simulink model "Catwell_Rom"  (R2023a)
settings: Solver=FixedStepDiscrete  StartTime=0.0  StopTime=3.999  FixedStep=.01  RelTol=1e-3
libraries: Pathfinding_lib x4, simulink x2, embmathops x1, dspsigops x1, drivinglib x1
settings Model: SimulationMode=accelerator  Creator=FIRSTMentor  LastModifiedBy=ander

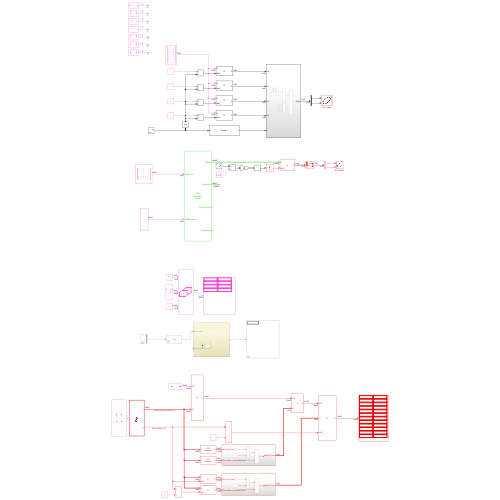
[thumbnail: Simulink's stored preview of the top-level diagram]
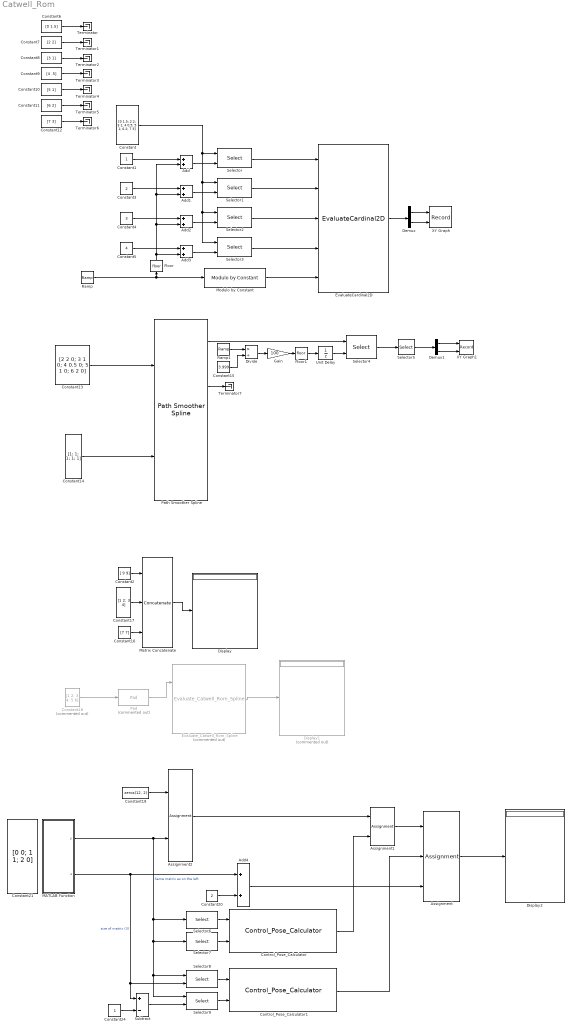
== system Catwell_Rom ==
  Add{,1..4} (5 alike) : Sum
  Assignment : Assignment  NumberOfDimensions=2  DiagnosticForDimensions=Warning  IndexOptions=Starting index (port),Assign all  Indices=1,1  OutputSizes=1,1
  Assignment1 : Assignment  NumberOfDimensions=2  DiagnosticForDimensions=Warning  IndexOptions=Starting index (dialog),Assign all  Indices=1,1  OutputSizes=1,1
  Assignment2 : Assignment  NumberOfDimensions=2  DiagnosticForDimensions=Warning  IndexOptions=Starting index (dialog),Assign all  Indices=2,2  OutputSizes=1,1
  Constant : Constant  Value=[0 1.5; 2 2; 3 1; 4 0.5; 5 1; 6 2; 7 3]  VectorParams1D=off
  Constant1 : Constant
  Constant10 : Constant  Value=[5 1]
  Constant11 : Constant  Value=[6 2]
  Constant12 : Constant  Value=[7 3]
  Constant13 : Constant  Value=[2 2 0; 3 1 0; 4 0.5 0; 5 1 0; 6 2 0]  VectorParams1D=off
  Constant14 : Constant  Value=[1; 1; 1; 1; 1]  VectorParams1D=off
  Constant15 : Constant  Value=3.999
  Constant16 : Constant  Value=[7 7]  VectorParams1D=off
  Constant17 : Constant  Value=[1 2; 3 4]  VectorParams1D=off
  Constant18 : Constant  Commented=on  Value=[1 2; 3 4; 5 6]
  Constant19 : Constant  Value=zeros(12, 2)
  Constant2 : Constant  Value=[ 9 9]  VectorParams1D=off
  Constant20 : Constant  Value=2
  Constant21 : Constant  Value=[0 0; 1 1; 2 0]
  Constant24 : Constant
  Constant3 : Constant  Value=2
  Constant4 : Constant  Value=3
  Constant5 : Constant  Value=4
  Constant6 : Constant  Value=[0 1.5]
  Constant7 : Constant  Value=[2 2]
  Constant8 : Constant  Value=[3 1]
  Constant9 : Constant  Value=[4 .5]
  Control_Pose_Calculator : Pathfinding_lib/Control_Pose_Calculator  SystemSampleTime=-1  VariantActivationTime=update diagram  Latency=0  AutoFrameSizeCalculation=off
  Control_Pose_Calculator1 : Pathfinding_lib/Control_Pose_Calculator  SystemSampleTime=-1  VariantActivationTime=update diagram  Latency=0  AutoFrameSizeCalculation=off
  Demux : Demux  Outputs=2
  Demux1 : Demux  Outputs=2
  Display : Display
  Display1 : Display  Commented=on
  Display2 : Display
  Divide : Product  Inputs=*/  RndMeth=Zero  SaturateOnIntegerOverflow=on
  EvaluateCardinal2D : Pathfinding_lib/EvaluateCardinal2D  SystemSampleTime=-1  VariantActivationTime=update diagram  Latency=0  AutoFrameSizeCalculation=off
  Evaluate_Catwell_Rom_Spline : Pathfinding_lib/Evaluate_Catwell_Rom_Spline  Commented=on  SystemSampleTime=-1  VariantActivationTime=update diagram  Latency=0  AutoFrameSizeCalculation=off
  Floor : Rounding
  Floor1 : Rounding
  Gain : Gain  Gain=100
  MATLAB Function : MATLAB Function  TreatAsAtomicUnit=on
  Matrix Concatenate : Concatenate  NumInputs=3  Mode=Multidimensional array
  Modulo by Constant : embmathops/Modulo by Constant  Denominator=1  SimulateUsing=Code generation
      settings: LibrarySourceBlock=embeddedMathLib/Modulo by Constant
  Pad : dspsigops/Pad  Commented=on  padAlong=Columns  dimsToPad=1  valSrc=Specify via dialog  padVal=-1  spec=Output size  padNumOutRowsSpecMethod=User-specified  numOutRows=Spline_Max_Num_RefPoses  padNumOutColsSpecMethod=User-specified  numOutCols=10  isVarDimsMode=off  padBeginning=0  padEnd=0  outSizeMode=User-specified  outSize=1  padSigAt=End  trunc_flag=None  roundingMode=Floor  overflowMode=off  truncOrWrapMode=Truncate  wrap_flag=None
  Path Smoother Spline : drivinglib/Path Smoother Spline  NumSmoothPoses=100  MinSeparation=1e-3  SampleTime=0.5  ShowOptionalOutports=on  SimulateUsing=Code generation
  Ramp : simulink/Sources/Ramp  slope=1  start=0  InitialOutput=0
  Ramp1 : simulink/Sources/Ramp  slope=1  start=0  InitialOutput=0
  Selector : Selector  NumberOfDimensions=2  InputPortWidth=7,2  IndexOptions=Index vector (port),Select all  Indices=[1],1  OutputSizes=1,1
  Selector1 : Selector  NumberOfDimensions=2  InputPortWidth=7  IndexOptions=Index vector (port),Select all  Indices=[2],1  OutputSizes=1,1
  Selector2 : Selector  NumberOfDimensions=2  InputPortWidth=7  IndexOptions=Index vector (port),Select all  Indices=[3],1  OutputSizes=1,1
  Selector3 : Selector  NumberOfDimensions=2  InputPortWidth=7  IndexOptions=Index vector (port),Select all  Indices=[4],1  OutputSizes=1,1
  Selector4 : Selector  NumberOfDimensions=2  IndexMode=Zero-based  InputPortWidth=3  IndexOptions=Index vector (port),Select all  Indices=[1 3],1  OutputSizes=1,1
  Selector5 : Selector  InputPortWidth=3  IndexOptions=Index vector (dialog)  Indices=[1 2]  OutputSizes=1
  Selector6 : Selector  NumberOfDimensions=2  InputPortWidth=3  IndexOptions=Index vector (dialog),Select all  Indices=[1],1  OutputSizes=1,1
  Selector7 : Selector  NumberOfDimensions=2  InputPortWidth=3  IndexOptions=Index vector (dialog),Select all  Indices=[2],1  OutputSizes=1,1
  Selector8 : Selector  NumberOfDimensions=2  InputPortWidth=3  IndexOptions=Index vector (port),Select all  Indices=[1],1  OutputSizes=1,1
  Selector9 : Selector  NumberOfDimensions=2  InputPortWidth=3  IndexOptions=Index vector (port),Select all  Indices=[2],1  OutputSizes=1,1
  Subtract : Sum  Inputs=+-
  Terminator{,1..7} (8 alike) : Terminator
  Unit Delay : UnitDelay  SampleTime=-1  HasFrameUpgradeWarning=on
  XY Graph : Record  FileSettingsInternal="{\"entries\":[{\"content\":{\"excelSettings\":{\"content\":{},\"type\":\"Streamout.ExcelSettings\"}},\"type\":\"Streamout.FileSettingStorage\",\"uuid\":\"\"}],\"packageUris\":[\"http:\\/\\/schema.mathworks.com\\/mf0\\/streamout_blocks\\/R2020a\"],\"version\":\"1.0\"}"  Layout=[1 1]  SignalsInternal="{\"entries\":[{\"content\":{\"signals\":[{\"content\":{\"blockPath\":[],\"dimensions\":[1,1],\"domain\":\"\",\"lineColor\":\"#a2142f\",\"plots\":[1],\"port\":1,\"sid\":[\"\"],\"signalID\":6505,\"signalName\":\"Demux:1\"},\"type\":\"RecordBlkView.Signal\",\"uuid\":\"\"},{\"content\":{\"blockPath\":[],\"dimensions\":[1,1],\"domain\":\"\",\"lineColor\":\"#139fff\",\"plots\":[1],\"port\":2,\"sid\":[\"\"],\"signalID\":6509,\"signalName\":\"Demux:2\"},\"type\":\"RecordBlkView.Signal\",\"uuid\":\"\"}]},\"type\":\"RecordBlkView.InputSignals\",\"uuid\":\"\"}],\"packageUris\":[\"http:\\/\\/schema.mathworks.com\\/mf0\\/streamout_blocks\\/R2020a\"],\"version\":\"1.0\"}"  VisualizationBindings="{\"xyplotplugin\":{\"info\":[{\"series\":[{\"bindingParametersList\":[{\"parameter\":\"X-Axis\",\"signalID\":6505,\"signalName\":\"Demux:1\"},{\"parameter\":\"Y-Axis\",\"signalID\":6509,\"signalName\":\"Demux:2\"}],\"seriesID\":8380}],\"subplotID\":1}]}}"  CompatibilityTag=XY
  XY Graph1 : Record  FileSettingsInternal="{\"entries\":[{\"content\":{\"excelSettings\":{\"content\":{},\"type\":\"Streamout.ExcelSettings\"}},\"type\":\"Streamout.FileSettingStorage\",\"uuid\":\"\"}],\"packageUris\":[\"http:\\/\\/schema.mathworks.com\\/mf0\\/streamout_blocks\\/R2020a\"],\"version\":\"1.0\"}"  Layout=[1 1]  SignalsInternal="{\"entries\":[{\"content\":{\"signals\":[{\"content\":{\"blockPath\":[],\"dimensions\":[1,1],\"domain\":\"\",\"lineColor\":\"#a2142f\",\"plots\":[1],\"port\":1,\"sid\":[\"\"],\"signalID\":6513,\"signalName\":\"Demux1:1\"},\"type\":\"RecordBlkView.Signal\",\"uuid\":\"\"},{\"content\":{\"blockPath\":[],\"dimensions\":[1,1],\"domain\":\"\",\"lineColor\":\"#139fff\",\"plots\":[1],\"port\":2,\"sid\":[\"\"],\"signalID\":6517,\"signalName\":\"Demux1:2\"},\"type\":\"RecordBlkView.Signal\",\"uuid\":\"\"}]},\"type\":\"RecordBlkView.InputSignals\",\"uuid\":\"\"}],\"packageUris\":[\"http:\\/\\/schema.mathworks.com\\/mf0\\/streamout_blocks\\/R2020a\"],\"version\":\"1.0\"}"  VisualizationBindings="{\"xyplotplugin\":{\"info\":[{\"series\":[{\"bindingParametersList\":[{\"parameter\":\"X-Axis\",\"signalID\":6513,\"signalName\":\"Demux1:1\"},{\"parameter\":\"Y-Axis\",\"signalID\":6517,\"signalName\":\"Demux1:2\"}],\"seriesID\":22464}],\"subplotID\":1}]}}"  CompatibilityTag=XY
  wires:
  Ramp/1 -> Modulo by Constant/1, Floor/1
  Constant/1 -> Selector3/1, Selector2/1, Selector1/1, Selector/1
  Selector3/1 -> EvaluateCardinal2D/4
  Selector2/1 -> EvaluateCardinal2D/3
  Selector1/1 -> EvaluateCardinal2D/2
  Selector/1 -> EvaluateCardinal2D/1
  EvaluateCardinal2D/1 -> Demux/1
  Demux/1 -> XY Graph/1
  Demux/2 -> XY Graph/2
  Modulo by Constant/1 -> EvaluateCardinal2D/5
  Add/1 -> Selector/2
  Add1/1 -> Selector1/2
  Add2/1 -> Selector2/2
  Add3/1 -> Selector3/2
  Constant1/1 -> Add/1
  Constant3/1 -> Add1/1
  Constant4/1 -> Add2/1
  Constant5/1 -> Add3/1
  Floor/1 -> Add/2, Add1/2, Add2/2, Add3/2
  Constant12/1 -> Terminator6/1
  Constant11/1 -> Terminator5/1
  Constant10/1 -> Terminator4/1
  Constant9/1 -> Terminator3/1
  Constant8/1 -> Terminator2/1
  Constant7/1 -> Terminator1/1
  Constant6/1 -> Terminator/1
  Constant13/1 -> Path Smoother Spline/1
  Constant14/1 -> Path Smoother Spline/2
  Path Smoother Spline/2 -> Terminator7/1
  Path Smoother Spline/1 -> Selector4/1
  Floor1/1 -> Unit Delay/1
  Selector4/1 -> Selector5/1
  Selector5/1 -> Demux1/1
  Demux1/1 -> XY Graph1/1
  Demux1/2 -> XY Graph1/2
  Ramp1/1 -> Divide/1
  Constant15/1 -> Divide/2
  Divide/1 -> Gain/1
  Gain/1 -> Floor1/1
  Unit Delay/1 -> Selector4/2
  Constant2/1 -> Matrix Concatenate/1
  Constant17/1 -> Matrix Concatenate/2
  Constant16/1 -> Matrix Concatenate/3
  Matrix Concatenate/1 -> Display/1
  Constant18/1 -> Pad/1
  Evaluate_Catwell_Rom_Spline/1 -> Display1/1
  Pad/1 -> Evaluate_Catwell_Rom_Spline/1
  MATLAB Function/1(y) -> Selector7/1, Selector9/1, Selector8/1, Selector6/1, Assignment2/2  "Same matrix as on the left"
  Constant19/1 -> Assignment2/1
  Assignment2/1 -> Assignment1/1
  Assignment1/1 -> Assignment/1
  MATLAB Function/2(s) -> Add4/1, Selector8/2, Subtract/1  "size of matrix (3)"
  Add4/1 -> Assignment/3
  Constant20/1 -> Add4/2
  Assignment/1 -> Display2/1
  Selector6/1 -> Control_Pose_Calculator/1
  Selector7/1 -> Control_Pose_Calculator/2
  Selector9/1 -> Control_Pose_Calculator1/2
  Selector8/1 -> Control_Pose_Calculator1/1
  Subtract/1 -> Selector9/2
  Constant24/1 -> Subtract/2
  Control_Pose_Calculator/1 -> Assignment1/2
  Control_Pose_Calculator1/1 -> Assignment/2

== matlab function Catwell_Rom/MATLAB Function ==
  data: y output size=[10 2]; s output
function [y, s] = fcn()
y = [1 2; 3 4; 5 6; 7 8];
s = 4;
end
